simulink model "PID"  (R2016b)
settings: Solver=FixedStepAuto  StartTime=0.0  StopTime=10.0  FixedStep=0.01  RelTol=1e-3
values from neighbouring files (symbols this model uses):
  den = [1 0.1313 1.109]    [UpdatedSimulinkValues-2.m]    (also in UpdatedSimulinkValuesalex1.m; part2a.m)
  num = [0.26*1.109*180/pi()]    [UpdatedSimulinkValues-2.m]    (also in UpdatedSimulinkValuesalex1.m; part2a.m)
undefined symbols (not defined in the file or in its folder): G
settings Model: Creator=Akash  LastModifiedBy=Akash
settings SolverCC: MaxConsecutiveMinStep=2

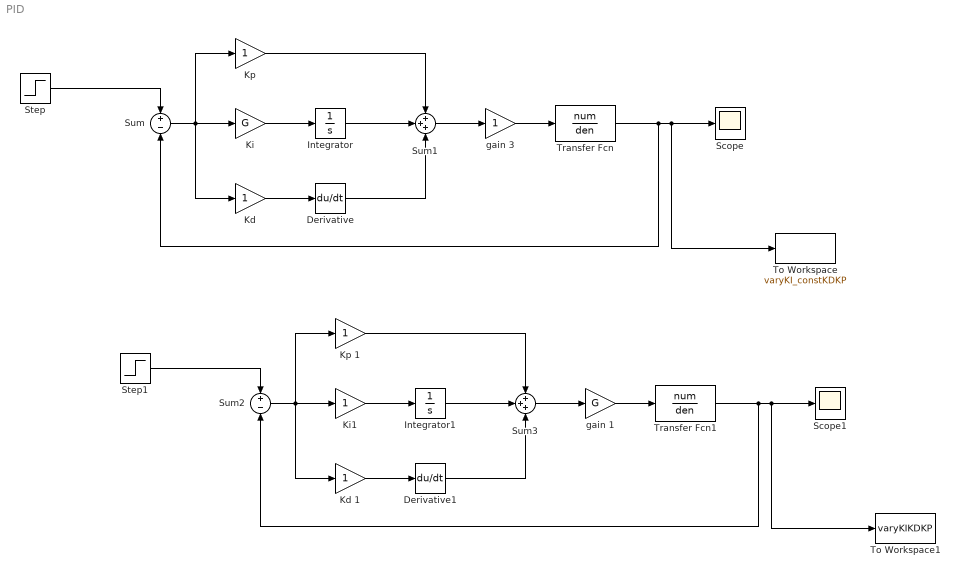
== system PID ==
  Derivative : Derivative
  Derivative1 : Derivative
  Integrator : Integrator
  Integrator1 : Integrator
  "Kd " : Gain
  Kd 1 : Gain
  Ki : Gain  Gain=G
  Ki1 : Gain
  "Kp " : Gain
  Kp 1 : Gain
  Scope : Scope
  Scope1 : Scope
  Step : Step  SampleTime=0
  Step1 : Step  SampleTime=0
  Sum : Sum  Inputs=+-
  Sum1 : Sum  Inputs=+++
  Sum2 : Sum  Inputs=+-
  Sum3 : Sum  Inputs=+++
  To Workspace : ToWorkspace  VariableName=varyKI_constKDKP  SaveFormat=Timeseries  SampleTime=-1
  To Workspace1 : ToWorkspace  VariableName=varyKIKDKP  SaveFormat=Timeseries  SampleTime=-1
  Transfer Fcn : TransferFcn  Numerator=num  Denominator=den
  Transfer Fcn1 : TransferFcn  Numerator=num  Denominator=den
  gain 1 : Gain  Gain=G
  gain 3 : Gain
  wires:
  Transfer Fcn/1 -> Scope/1, To Workspace/1, Sum/2
  Step/1 -> Sum/1
  Sum/1 -> "Kp "/1, "Kd "/1, Ki/1
  Ki/1 -> Integrator/1
  Integrator/1 -> Sum1/2
  "Kd "/1 -> Derivative/1
  Derivative/1 -> Sum1/3
  "Kp "/1 -> Sum1/1
  Sum1/1 -> gain 3/1
  gain 3/1 -> Transfer Fcn/1
  Transfer Fcn1/1 -> Scope1/1, To Workspace1/1, Sum2/2
  Step1/1 -> Sum2/1
  Sum2/1 -> Kp 1/1, Kd 1/1, Ki1/1
  Ki1/1 -> Integrator1/1
  Integrator1/1 -> Sum3/2
  Kd 1/1 -> Derivative1/1
  Derivative1/1 -> Sum3/3
  Kp 1/1 -> Sum3/1
  Sum3/1 -> gain 1/1
  gain 1/1 -> Transfer Fcn1/1
